simulink model "simulationModel"  (R2024b)
settings: Solver=FixedStepDiscrete  StartTime=0.0  StopTime=4  RelTol=1e-3
libraries: dspvision x8, deeplib x1, audioai x1
settings Model: Creator=dhruva  LastModifiedBy=dhruva
settings SolverCC: AlgebraicLoopSolver=TrustRegion  AutoInsertRateTranBlk=on
settings DataIOCC: LimitDataPoints=on  SaveOutput=off  SignalLogging=off  SaveTime=off
settings OptimizationCC: LifeSpan=inf
settings DebuggingCC: AlgebraicLoopMsg=error  SingleTaskRateTransMsg=error  UnconnectedInputMsg=warning  UnconnectedOutputMsg=warning  UnconnectedLineMsg=warning  AllowSymbolicDim=off  SFUnexpectedBacktrackingDiag=warning  SFNoUnconditionalDefaultTransitionDiag=warning  SFExecutionAtInitializationDiag=none  ArithmeticOperatorsInVariantConditions=warning
settings ModelReferenceCC: EnableRefExpFcnMdlSchedulingChecks=on
settings SFSimCC: SimUseLocalCustomCode=off  CustomCodeUndefinedFunction=UseInterfaceOnly
settings RTWCC: RTWUseLocalCustomCode=off  GPUComputeCapability=3.5
settings CodeAppCC: StateflowObjectComments=on
settings GRTTargetCC: TargetLangStandard=C89/C90 (ANSI)
settings ConfigComp: CovMetricSettings=dw  CovSaveCumulativeToWorkspaceVar=on  CovSaveSingleToWorkspaceVar=on  CovExternalEMLEnable=off  CovSFcnEnable=off

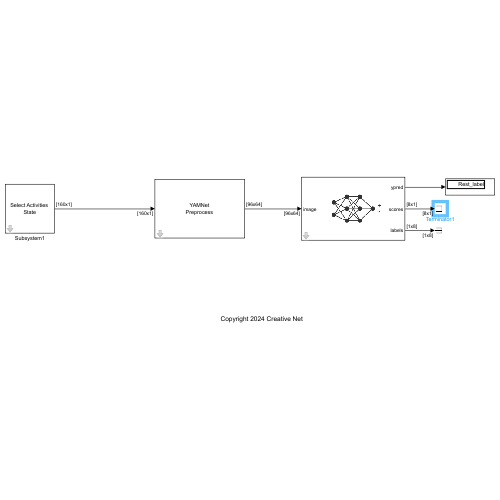
[thumbnail: Simulink's stored preview of the top-level diagram]
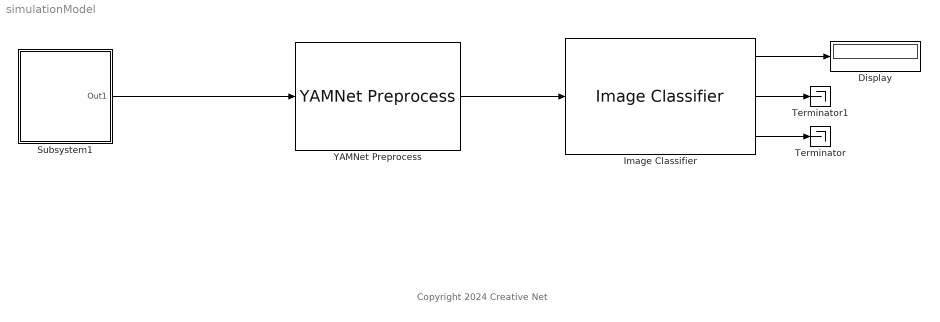
== system simulationModel ==
  note: Copyright 2024 Creative Net
  Display : Display
  Image Classifier : deeplib/Image Classifier  Network=Network from MAT-file  NetworkFunction=squeezenet  NetworkFilePath=D:\projects\Research\Mind Control Bionic Arm\Models\Direct Brainwave Signal\graded learning\model.mat  NetworkClassesVariable=classNames  MiniBatchSize=128  ResizeInput=on  Classification=on  Predictions=on  ForceInterpretedSim=off  PredictMode=All probabilities and labels  K=5
  Subsystem1 : Subsystem  mask{SoundType=BEO}
      mask prompts: SoundType "Type"
      mask init:
      | t = get_param(gcb,'SoundType');
      | 
      | val = 1;
      | switch t
      |     case {'BEO'}
      |         val = 1;
      |     case {'CLH'}
      |         val = 2;
      |     case {'CRH'}
      |         val = 3;
      |     case {'DLF'}
      |         val = 4;
      |     case {'DRF'}
      |         val = 5;
      |     case {'PLF'}
      |         val = 6;
      |     case {'PRF'}
      |         val = 7;
      |     case {'Rest'}
      |         val = 8;
      | end
      | 
      | set_param([gcb '/Constant'],'Value',num2str(val));
      mask TypeOptions SoundType: BEO | CLH | CRH | DLF | DRF | PLF | PRF | Rest
      mask Display: fprintf('Select Activities \nState')
  Terminator : Terminator
  Terminator1 : Terminator
  YAMNet Preprocess : audioai/YAMNet Preprocess  InputSampleRate=16e3  OverlapPercent=50
  wires:
  Subsystem1/1(Out1) -> YAMNet Preprocess/1
  YAMNet Preprocess/1 -> Image Classifier/1
  Image Classifier/1 -> Display/1
  Image Classifier/2 -> Terminator1/1
  Image Classifier/3 -> Terminator/1

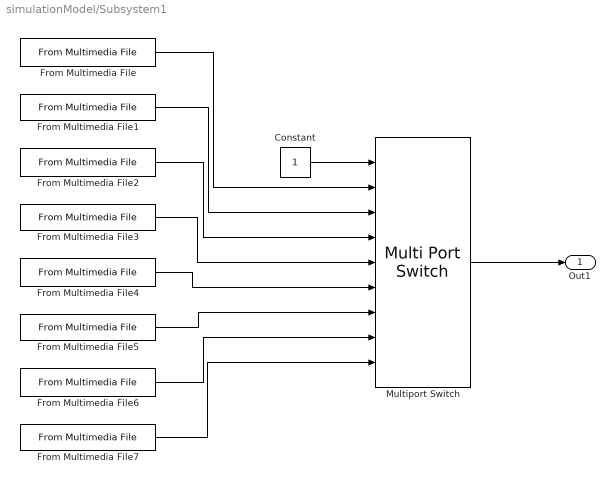
== system simulationModel/Subsystem1 ==
  Constant : Constant
  From Multimedia File : dspvision/From Multimedia File  inputFilename=D:\projects\Research\Mind Control Bionic Arm\datasets\audioFiles\BEO\BEO_1_0.wav  readRange=[1 Inf]  loop=on  numPlays=1  outputStreams=Audio only  videoDataType=single  audioDataType=double  inheritSampleTime=on  userDefinedSampleTime=1/30  noAudioOutput=off  isIntensityVideo=off  fourcc=RGB  colorVideoFormat=Separate color signals  outputEOF=off  dataOrg=Column-major  audioFrameSize=160  computeAudioFrameSize=off  outSamplingMode=Sample based
  From Multimedia File1 : dspvision/From Multimedia File  inputFilename=D:\projects\Research\Mind Control Bionic Arm\datasets\audioFiles\CLH\CLH_100_0.wav  readRange=[1 Inf]  loop=on  numPlays=1  outputStreams=Audio only  videoDataType=single  audioDataType=double  inheritSampleTime=on  userDefinedSampleTime=1/30  noAudioOutput=off  isIntensityVideo=off  fourcc=RGB  colorVideoFormat=Separate color signals  outputEOF=off  dataOrg=Column-major  audioFrameSize=160  computeAudioFrameSize=off  outSamplingMode=Sample based
  From Multimedia File2 : dspvision/From Multimedia File  inputFilename=D:\projects\Research\Mind Control Bionic Arm\datasets\audioFiles\CRH\CRH_100_0.wav  readRange=[1 Inf]  loop=on  numPlays=1  outputStreams=Audio only  videoDataType=single  audioDataType=double  inheritSampleTime=on  userDefinedSampleTime=1/30  noAudioOutput=off  isIntensityVideo=off  fourcc=RGB  colorVideoFormat=Separate color signals  outputEOF=off  dataOrg=Column-major  audioFrameSize=160  computeAudioFrameSize=off  outSamplingMode=Sample based
  From Multimedia File3 : dspvision/From Multimedia File  inputFilename=D:\projects\Research\Mind Control Bionic Arm\datasets\audioFiles\DLF\DLF_100_0.wav  readRange=[1 Inf]  loop=on  numPlays=1  outputStreams=Audio only  videoDataType=single  audioDataType=double  inheritSampleTime=on  userDefinedSampleTime=1/30  noAudioOutput=off  isIntensityVideo=off  fourcc=RGB  colorVideoFormat=Separate color signals  outputEOF=off  dataOrg=Column-major  audioFrameSize=160  computeAudioFrameSize=off  outSamplingMode=Sample based
  From Multimedia File4 : dspvision/From Multimedia File  inputFilename=D:\projects\Research\Mind Control Bionic Arm\datasets\audioFiles\DRF\DRF_100_0.wav  readRange=[1 Inf]  loop=on  numPlays=1  outputStreams=Audio only  videoDataType=single  audioDataType=double  inheritSampleTime=on  userDefinedSampleTime=1/30  noAudioOutput=off  isIntensityVideo=off  fourcc=RGB  colorVideoFormat=Separate color signals  outputEOF=off  dataOrg=Column-major  audioFrameSize=160  computeAudioFrameSize=off  outSamplingMode=Sample based
  From Multimedia File5 : dspvision/From Multimedia File  inputFilename=D:\projects\Research\Mind Control Bionic Arm\datasets\audioFiles\PLF\PLF_100_0.wav  readRange=[1 Inf]  loop=on  numPlays=1  outputStreams=Audio only  videoDataType=single  audioDataType=double  inheritSampleTime=on  userDefinedSampleTime=1/30  noAudioOutput=off  isIntensityVideo=off  fourcc=RGB  colorVideoFormat=Separate color signals  outputEOF=off  dataOrg=Column-major  audioFrameSize=160  computeAudioFrameSize=off  outSamplingMode=Sample based
  From Multimedia File6 : dspvision/From Multimedia File  inputFilename=D:\projects\Research\Mind Control Bionic Arm\datasets\audioFiles\PRF\PRF_100_0.wav  readRange=[1 Inf]  loop=on  numPlays=1  outputStreams=Audio only  videoDataType=single  audioDataType=double  inheritSampleTime=on  userDefinedSampleTime=1/30  noAudioOutput=off  isIntensityVideo=off  fourcc=RGB  colorVideoFormat=Separate color signals  outputEOF=off  dataOrg=Column-major  audioFrameSize=160  computeAudioFrameSize=off  outSamplingMode=Sample based
  From Multimedia File7 : dspvision/From Multimedia File  inputFilename=D:\projects\Research\Mind Control Bionic Arm\datasets\audioFiles\Rest\Rest_1000_0.wav  readRange=[1 Inf]  loop=on  numPlays=1  outputStreams=Audio only  videoDataType=single  audioDataType=double  inheritSampleTime=on  userDefinedSampleTime=1/30  noAudioOutput=off  isIntensityVideo=off  fourcc=RGB  colorVideoFormat=Separate color signals  outputEOF=off  dataOrg=Column-major  audioFrameSize=160  computeAudioFrameSize=off  outSamplingMode=Sample based
  Multiport Switch : MultiPortSwitch  Inputs=8  SaturateOnIntegerOverflow=off  InputSameDT=off
  Out1 : Outport
  wires:
  From Multimedia File2/1 -> Multiport Switch/4
  From Multimedia File/1 -> Multiport Switch/2
  From Multimedia File6/1 -> Multiport Switch/8
  From Multimedia File3/1 -> Multiport Switch/5
  From Multimedia File4/1 -> Multiport Switch/6
  From Multimedia File1/1 -> Multiport Switch/3
  From Multimedia File5/1 -> Multiport Switch/7
  From Multimedia File7/1 -> Multiport Switch/9
  Constant/1 -> Multiport Switch/1
  Multiport Switch/1 -> Out1/1
